simulink model "pmsm_observer_pll_block_model"  (R2024b)
settings: Solver=FixedStepDiscrete  StartTime=0.0  StopTime=0.15  FixedStep=Ts  RelTol=1e-3
InitFcn:
  | model_file = get_param(bdroot, 'FileName');
  | model_dir = fileparts(model_file);
  | run(fullfile(model_dir, 'pmsm_observer_pll_params.m'));
values from neighbouring files (symbols this model uses):
  flux_limit = flux_wb * flux_limit_ratio    (= 0.0117)    [pmsm_observer_pll_params.m]
  flux_wb = 0.0078    [pmsm_observer_pll_params.m]
  Ld = Ls    (= 0.0006)    [pmsm_observer_pll_params.m]
  Lq = Ls    (= 0.0006)    [pmsm_observer_pll_params.m]
  Ls = 0.0006    [pmsm_observer_pll_params.m]
  obs_eps = 1.0e-6    (= 1e-06)    [pmsm_observer_pll_params.m]
  obs_speed_filter_alpha = 0.05    [pmsm_observer_pll_params.m]
  obs_speed_limit_rad_s = 2200.0    (= 2200)    [pmsm_observer_pll_params.m]
  obs_theta_comp_rad = 2.2003    [pmsm_observer_pll_params.m]
  pll_integral_limit = 1800.0    (= 1800)    [pmsm_observer_pll_params.m]
  pll_ki = 3000.0    (= 3000)    [pmsm_observer_pll_params.m]
  pll_kp = 120.0    (= 120)    [pmsm_observer_pll_params.m]
  pole_pairs = 4.0    (= 4)    [pmsm_observer_pll_params.m]
  Rs = 0.53    [pmsm_observer_pll_params.m]
  sim_id_a = 0.0    (= 0)    [pmsm_observer_pll_params.m]
  sim_iq_a = 1.0    (= 1)    [pmsm_observer_pll_params.m]
  sim_mech_speed_rad_s = 2000.0 * 2.0 * pi / 60.0    (= 209.439510239)    [pmsm_observer_pll_params.m]
  Ts = 6.25e-5    (= 6.25e-05)    [pmsm_observer_pll_params.m]
undefined symbols (not defined in the file or in its folder): DiscIntNeverNeededParam
settings Model: Creator=10095  LastModifiedBy=10095
settings DataIOCC: SaveFormat=StructureWithTime

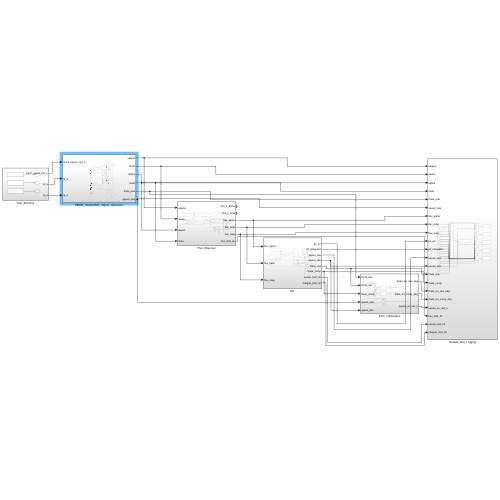
[thumbnail: Simulink's stored preview of the top-level diagram]
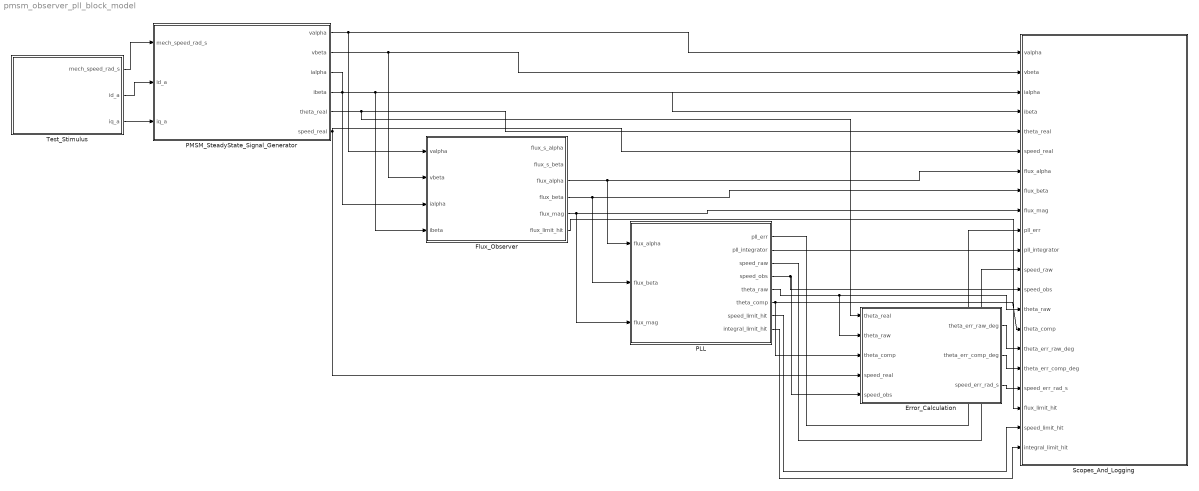
== system pmsm_observer_pll_block_model ==
  Error_Calculation : Subsystem
  Flux_Observer : Subsystem
  PLL : Subsystem
  PMSM_SteadyState_Signal_Generator : Subsystem
  Scopes_And_Logging : Subsystem
  Test_Stimulus : Subsystem
  wires:
  Test_Stimulus/3(iq_a) -> PMSM_SteadyState_Signal_Generator/3(iq_a)
  PLL/6(theta_comp) -> Error_Calculation/3(theta_comp), Scopes_And_Logging/15(theta_comp)
  PLL/2(pll_integrator) -> Scopes_And_Logging/11(pll_integrator)
  Flux_Observer/4(flux_beta) -> Scopes_And_Logging/8(flux_beta), PLL/2(flux_beta)
  Test_Stimulus/1(mech_speed_rad_s) -> PMSM_SteadyState_Signal_Generator/1(mech_speed_rad_s)
  Test_Stimulus/2(id_a) -> PMSM_SteadyState_Signal_Generator/2(id_a)
  PMSM_SteadyState_Signal_Generator/5(theta_real) -> Error_Calculation/1(theta_real), Scopes_And_Logging/5(theta_real)
  PMSM_SteadyState_Signal_Generator/4(ibeta) -> Scopes_And_Logging/4(ibeta), Flux_Observer/4(ibeta)
  PMSM_SteadyState_Signal_Generator/3(ialpha) -> Scopes_And_Logging/3(ialpha), Flux_Observer/3(ialpha)
  Error_Calculation/1(theta_err_raw_deg) -> Scopes_And_Logging/16(theta_err_raw_deg)
  PMSM_SteadyState_Signal_Generator/2(vbeta) -> Scopes_And_Logging/2(vbeta), Flux_Observer/2(vbeta)
  PMSM_SteadyState_Signal_Generator/1(valpha) -> Scopes_And_Logging/1(valpha), Flux_Observer/1(valpha)
  PMSM_SteadyState_Signal_Generator/6(speed_real) -> Error_Calculation/4(speed_real), Scopes_And_Logging/6(speed_real)
  PLL/7(speed_limit_hit) -> Scopes_And_Logging/20(speed_limit_hit)
  PLL/3(speed_raw) -> Scopes_And_Logging/12(speed_raw)
  Flux_Observer/3(flux_alpha) -> Scopes_And_Logging/7(flux_alpha), PLL/1(flux_alpha)
  PLL/5(theta_raw) -> Scopes_And_Logging/14(theta_raw), Error_Calculation/2(theta_raw)
  PLL/1(pll_err) -> Scopes_And_Logging/10(pll_err)
  Flux_Observer/5(flux_mag) -> Scopes_And_Logging/9(flux_mag), PLL/3(flux_mag)
  Flux_Observer/6(flux_limit_hit) -> Scopes_And_Logging/19(flux_limit_hit)
  PLL/4(speed_obs) -> Scopes_And_Logging/13(speed_obs), Error_Calculation/5(speed_obs)
  PLL/8(integral_limit_hit) -> Scopes_And_Logging/21(integral_limit_hit)
  Error_Calculation/2(theta_err_comp_deg) -> Scopes_And_Logging/17(theta_err_comp_deg)
  Error_Calculation/3(speed_err_rad_s) -> Scopes_And_Logging/18(speed_err_rad_s)

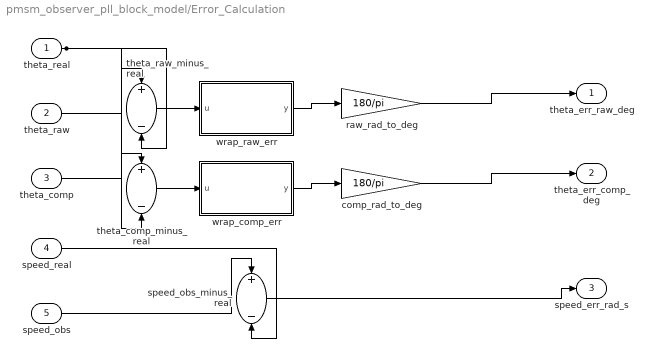
== system pmsm_observer_pll_block_model/Error_Calculation ==
  theta_real : Inport
  theta_raw : Inport  Port=2
  theta_comp : Inport  Port=3
  speed_real : Inport  Port=4
  speed_obs : Inport  Port=5
  comp_rad_to_deg : Gain  Gain=180/pi
  raw_rad_to_deg : Gain  Gain=180/pi
  speed_obs_minus_real : Sum  Inputs=+-
  theta_comp_minus_real : Sum  Inputs=+-
  theta_raw_minus_real : Sum  Inputs=+-
  wrap_comp_err : MATLAB Function  TreatAsAtomicUnit=on
  wrap_raw_err : MATLAB Function  TreatAsAtomicUnit=on
  theta_err_raw_deg : Outport
  theta_err_comp_deg : Outport  Port=2
  speed_err_rad_s : Outport  Port=3
  wires:
  theta_raw/1 -> theta_raw_minus_real/1
  theta_real/1 -> theta_raw_minus_real/2, theta_comp_minus_real/2
  theta_raw_minus_real/1 -> wrap_raw_err/1(u)
  wrap_raw_err/1(y) -> raw_rad_to_deg/1
  raw_rad_to_deg/1 -> theta_err_raw_deg/1
  theta_comp/1 -> theta_comp_minus_real/1
  theta_comp_minus_real/1 -> wrap_comp_err/1(u)
  wrap_comp_err/1(y) -> comp_rad_to_deg/1
  comp_rad_to_deg/1 -> theta_err_comp_deg/1
  speed_obs/1 -> speed_obs_minus_real/1
  speed_real/1 -> speed_obs_minus_real/2
  speed_obs_minus_real/1 -> speed_err_rad_s/1

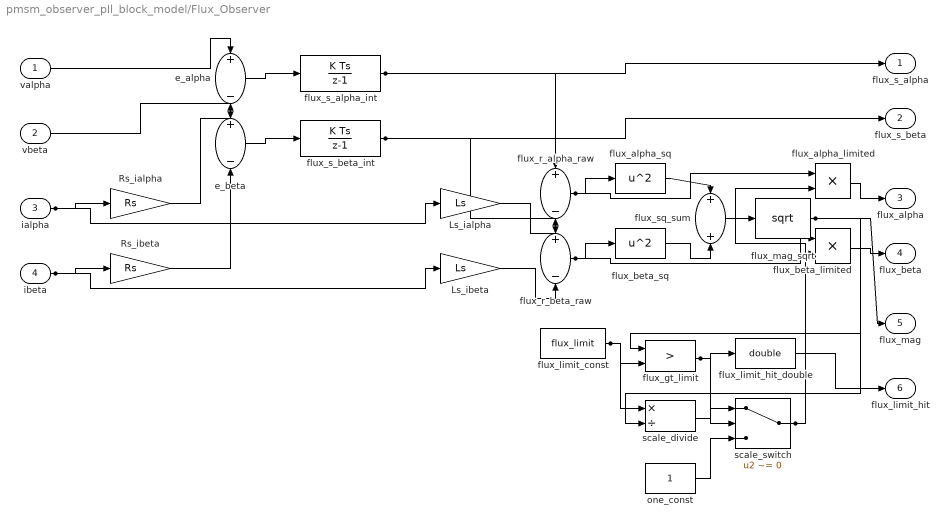
== system pmsm_observer_pll_block_model/Flux_Observer ==
  valpha : Inport
  vbeta : Inport  Port=2
  ialpha : Inport  Port=3
  ibeta : Inport  Port=4
  Ls_ialpha : Gain  Gain=Ls
  Ls_ibeta : Gain  Gain=Ls
  Rs_ialpha : Gain  Gain=Rs
  Rs_ibeta : Gain  Gain=Rs
  e_alpha : Sum  Inputs=+-
  e_beta : Sum  Inputs=+-
  flux_alpha_limited : Product
  flux_alpha_sq : Math  Operator=square
  flux_beta_limited : Product
  flux_beta_sq : Math  Operator=square
  flux_gt_limit : RelationalOperator  Operator=>  OutDataTypeStr=boolean  RndMeth=Simplest  InputSameDT=off
  flux_limit_const : Constant  Value=flux_limit
  flux_limit_hit_double : DataTypeConversion  OutDataTypeStr=double  SaturateOnIntegerOverflow=off  RndMeth=Floor
  flux_mag_sqrt : Math  Operator=sqrt
  flux_r_alpha_raw : Sum  Inputs=+-
  flux_r_beta_raw : Sum  Inputs=+-
  flux_s_alpha_int : DiscreteIntegrator  InitialCondition=flux_wb  SampleTime=Ts  ICPrevOutput=DiscIntNeverNeededParam  ICPrevScaledInput=DiscIntNeverNeededParam
  flux_s_beta_int : DiscreteIntegrator  SampleTime=Ts  ICPrevOutput=DiscIntNeverNeededParam  ICPrevScaledInput=DiscIntNeverNeededParam
  flux_sq_sum : Sum
  one_const : Constant
  scale_divide : Product  Inputs=*/
  scale_switch : Switch  Criteria=u2 ~= 0  SaturateOnIntegerOverflow=off  InputSameDT=off
  flux_s_alpha : Outport
  flux_s_beta : Outport  Port=2
  flux_alpha : Outport  Port=3
  flux_beta : Outport  Port=4
  flux_mag : Outport  Port=5
  flux_limit_hit : Outport  Port=6
  wires:
  ialpha/1 -> Rs_ialpha/1, Ls_ialpha/1
  ibeta/1 -> Rs_ibeta/1, Ls_ibeta/1
  valpha/1 -> e_alpha/1
  Rs_ialpha/1 -> e_alpha/2
  vbeta/1 -> e_beta/1
  Rs_ibeta/1 -> e_beta/2
  e_alpha/1 -> flux_s_alpha_int/1
  e_beta/1 -> flux_s_beta_int/1
  flux_s_alpha_int/1 -> flux_s_alpha/1, flux_r_alpha_raw/1
  flux_s_beta_int/1 -> flux_s_beta/1, flux_r_beta_raw/1
  Ls_ialpha/1 -> flux_r_alpha_raw/2
  Ls_ibeta/1 -> flux_r_beta_raw/2
  flux_r_alpha_raw/1 -> flux_alpha_sq/1, flux_alpha_limited/1
  flux_r_beta_raw/1 -> flux_beta_sq/1, flux_beta_limited/1
  flux_alpha_sq/1 -> flux_sq_sum/1
  flux_beta_sq/1 -> flux_sq_sum/2
  flux_sq_sum/1 -> flux_mag_sqrt/1
  flux_mag_sqrt/1 -> flux_mag/1, flux_gt_limit/1, scale_divide/2
  flux_limit_const/1 -> flux_gt_limit/2, scale_divide/1
  flux_gt_limit/1 -> flux_limit_hit_double/1, scale_switch/2
  flux_limit_hit_double/1 -> flux_limit_hit/1
  scale_divide/1 -> scale_switch/1
  one_const/1 -> scale_switch/3
  scale_switch/1 -> flux_alpha_limited/2, flux_beta_limited/2
  flux_alpha_limited/1 -> flux_alpha/1
  flux_beta_limited/1 -> flux_beta/1

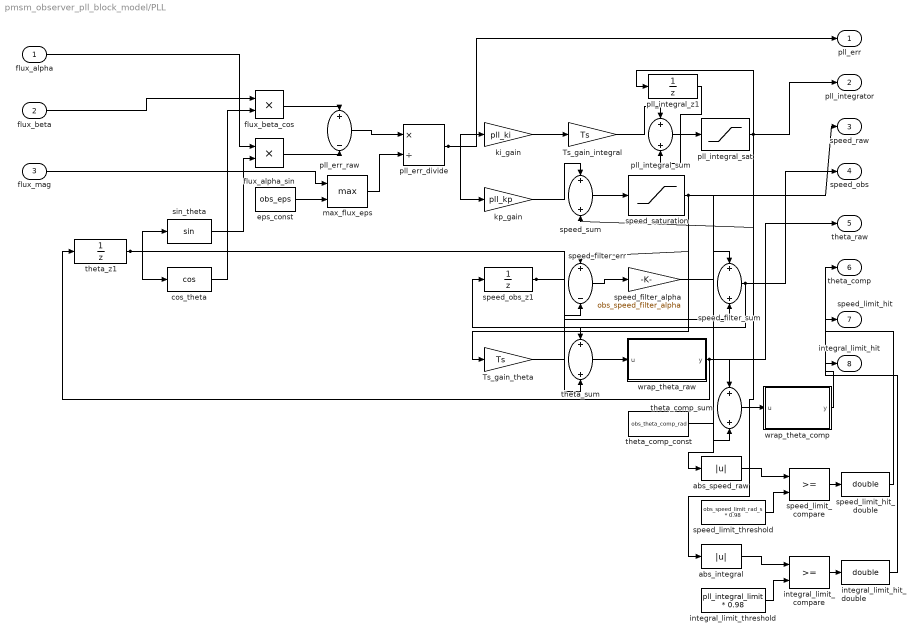
== system pmsm_observer_pll_block_model/PLL ==
  flux_alpha : Inport
  flux_beta : Inport  Port=2
  flux_mag : Inport  Port=3
  Ts_gain_integral : Gain  Gain=Ts
  Ts_gain_theta : Gain  Gain=Ts
  abs_integral : Abs  SaturateOnIntegerOverflow=off
  abs_speed_raw : Abs  SaturateOnIntegerOverflow=off
  cos_theta : Trigonometry  Operator=cos
  eps_const : Constant  Value=obs_eps
  flux_alpha_sin : Product
  flux_beta_cos : Product
  integral_limit_compare : RelationalOperator  OutDataTypeStr=boolean  RndMeth=Simplest  InputSameDT=off
  integral_limit_hit_double : DataTypeConversion  OutDataTypeStr=double  SaturateOnIntegerOverflow=off  RndMeth=Floor
  integral_limit_threshold : Constant  Value=pll_integral_limit * 0.98
  ki_gain : Gain  Gain=pll_ki
  kp_gain : Gain  Gain=pll_kp
  max_flux_eps : MinMax  Function=max  Inputs=2
  pll_err_divide : Product  Inputs=*/
  pll_err_raw : Sum  Inputs=+-
  pll_integral_sat : Saturate  UpperLimit=pll_integral_limit  LowerLimit=-pll_integral_limit
  pll_integral_sum : Sum
  pll_integral_z1 : UnitDelay  SampleTime=Ts  HasFrameUpgradeWarning=on
  sin_theta : Trigonometry
  speed_filter_alpha : Gain  Gain=obs_speed_filter_alpha
  speed_filter_err : Sum  Inputs=+-
  speed_filter_sum : Sum
  speed_limit_compare : RelationalOperator  OutDataTypeStr=boolean  RndMeth=Simplest  InputSameDT=off
  speed_limit_hit_double : DataTypeConversion  OutDataTypeStr=double  SaturateOnIntegerOverflow=off  RndMeth=Floor
  speed_limit_threshold : Constant  Value=obs_speed_limit_rad_s * 0.98
  speed_obs_z1 : UnitDelay  SampleTime=Ts  HasFrameUpgradeWarning=on
  speed_saturation : Saturate  UpperLimit=obs_speed_limit_rad_s  LowerLimit=-obs_speed_limit_rad_s
  speed_sum : Sum
  theta_comp_const : Constant  Value=obs_theta_comp_rad
  theta_comp_sum : Sum
  theta_sum : Sum
  theta_z1 : UnitDelay  SampleTime=Ts  HasFrameUpgradeWarning=on
  wrap_theta_comp : MATLAB Function  TreatAsAtomicUnit=on
  wrap_theta_raw : MATLAB Function  TreatAsAtomicUnit=on
  pll_err : Outport
  pll_integrator : Outport  Port=2
  speed_raw : Outport  Port=3
  speed_obs : Outport  Port=4
  theta_raw : Outport  Port=5
  theta_comp : Outport  Port=6
  speed_limit_hit : Outport  Port=7
  integral_limit_hit : Outport  Port=8
  wires:
  theta_z1/1 -> sin_theta/1, cos_theta/1, theta_sum/2
  flux_beta/1 -> flux_beta_cos/1
  cos_theta/1 -> flux_beta_cos/2
  flux_alpha/1 -> flux_alpha_sin/1
  sin_theta/1 -> flux_alpha_sin/2
  flux_beta_cos/1 -> pll_err_raw/1
  flux_alpha_sin/1 -> pll_err_raw/2
  flux_mag/1 -> max_flux_eps/1
  eps_const/1 -> max_flux_eps/2
  pll_err_raw/1 -> pll_err_divide/1
  max_flux_eps/1 -> pll_err_divide/2
  pll_err_divide/1 -> pll_err/1, ki_gain/1, kp_gain/1
  ki_gain/1 -> Ts_gain_integral/1
  Ts_gain_integral/1 -> pll_integral_sum/1
  pll_integral_z1/1 -> pll_integral_sum/2
  pll_integral_sum/1 -> pll_integral_sat/1
  pll_integral_sat/1 -> pll_integral_z1/1, pll_integrator/1, speed_sum/2, abs_integral/1
  kp_gain/1 -> speed_sum/1
  speed_sum/1 -> speed_saturation/1
  speed_saturation/1 -> speed_raw/1, speed_filter_err/1, Ts_gain_theta/1, abs_speed_raw/1
  speed_obs_z1/1 -> speed_filter_err/2, speed_filter_sum/2
  speed_filter_err/1 -> speed_filter_alpha/1
  speed_filter_alpha/1 -> speed_filter_sum/1
  speed_filter_sum/1 -> speed_obs_z1/1, speed_obs/1
  Ts_gain_theta/1 -> theta_sum/1
  theta_sum/1 -> wrap_theta_raw/1(u)
  wrap_theta_raw/1(y) -> theta_z1/1, theta_raw/1, theta_comp_sum/1
  theta_comp_const/1 -> theta_comp_sum/2
  theta_comp_sum/1 -> wrap_theta_comp/1(u)
  wrap_theta_comp/1(y) -> theta_comp/1
  abs_speed_raw/1 -> speed_limit_compare/1
  speed_limit_threshold/1 -> speed_limit_compare/2
  speed_limit_compare/1 -> speed_limit_hit_double/1
  speed_limit_hit_double/1 -> speed_limit_hit/1
  abs_integral/1 -> integral_limit_compare/1
  integral_limit_threshold/1 -> integral_limit_compare/2
  integral_limit_compare/1 -> integral_limit_hit_double/1
  integral_limit_hit_double/1 -> integral_limit_hit/1

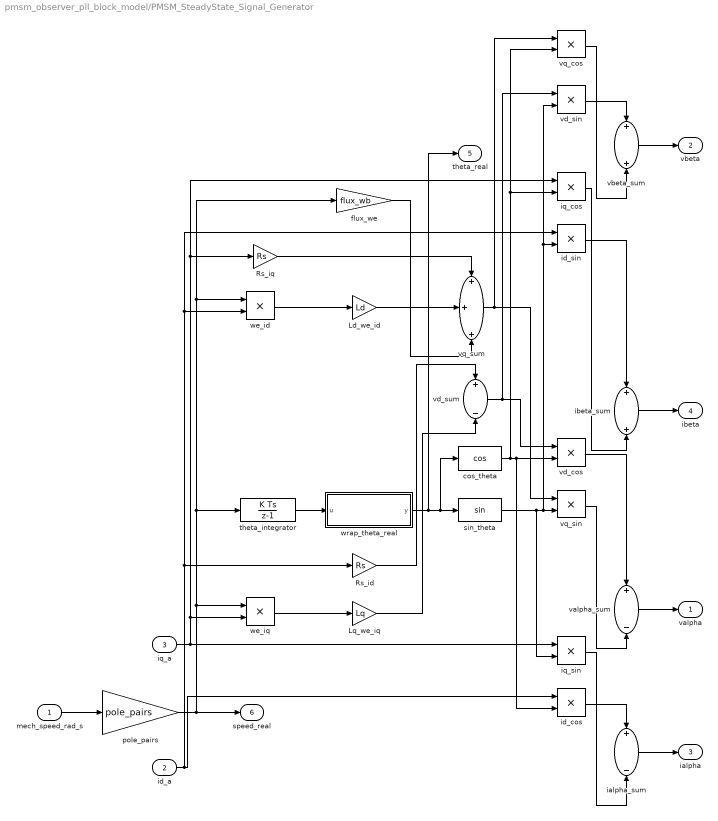
== system pmsm_observer_pll_block_model/PMSM_SteadyState_Signal_Generator ==
  mech_speed_rad_s : Inport
  id_a : Inport  Port=2
  iq_a : Inport  Port=3
  Ld_we_id : Gain  Gain=Ld
  Lq_we_iq : Gain  Gain=Lq
  Rs_id : Gain  Gain=Rs
  Rs_iq : Gain  Gain=Rs
  cos_theta : Trigonometry  Operator=cos
  flux_we : Gain  Gain=flux_wb
  ialpha_sum : Sum  Inputs=+-
  ibeta_sum : Sum
  id_cos : Product
  id_sin : Product
  iq_cos : Product
  iq_sin : Product
  pole_pairs : Gain  Gain=pole_pairs
  sin_theta : Trigonometry
  theta_integrator : DiscreteIntegrator  SampleTime=Ts  ICPrevOutput=DiscIntNeverNeededParam  ICPrevScaledInput=DiscIntNeverNeededParam
  valpha_sum : Sum  Inputs=+-
  vbeta_sum : Sum
  vd_cos : Product
  vd_sin : Product
  vd_sum : Sum  Inputs=+-
  vq_cos : Product
  vq_sin : Product
  vq_sum : Sum  Inputs=+++
  we_id : Product
  we_iq : Product
  wrap_theta_real : MATLAB Function  TreatAsAtomicUnit=on
  valpha : Outport
  vbeta : Outport  Port=2
  ialpha : Outport  Port=3
  ibeta : Outport  Port=4
  theta_real : Outport  Port=5
  speed_real : Outport  Port=6
  wires:
  id_a/1 -> id_sin/1, we_id/2, Rs_id/1, id_cos/1
  iq_a/1 -> Rs_iq/1, iq_cos/1, we_iq/2, iq_sin/1
  mech_speed_rad_s/1 -> pole_pairs/1
  vbeta_sum/1 -> vbeta/1
  vd_sin/1 -> vbeta_sum/1
  theta_integrator/1 -> wrap_theta_real/1(u)
  pole_pairs/1 -> flux_we/1, we_id/1, theta_integrator/1, we_iq/1, speed_real/1
  Rs_iq/1 -> vq_sum/1
  we_iq/1 -> Lq_we_iq/1
  we_id/1 -> Ld_we_id/1
  ibeta_sum/1 -> ibeta/1
  id_sin/1 -> ibeta_sum/1
  flux_we/1 -> vq_sum/3
  Ld_we_id/1 -> vq_sum/2
  vq_sin/1 -> valpha_sum/2
  vd_sum/1 -> vd_cos/1, vd_sin/1
  wrap_theta_real/1(y) -> cos_theta/1, sin_theta/1, theta_real/1
  Rs_id/1 -> vd_sum/1
  ialpha_sum/1 -> ialpha/1
  id_cos/1 -> ialpha_sum/1
  Lq_we_iq/1 -> vd_sum/2
  vq_cos/1 -> vbeta_sum/2
  vq_sum/1 -> vq_sin/1, vq_cos/1
  cos_theta/1 -> id_cos/2, vd_cos/2, iq_cos/2, vq_cos/2
  sin_theta/1 -> id_sin/2, vd_sin/2, vq_sin/2, iq_sin/2
  iq_cos/1 -> ibeta_sum/2
  valpha_sum/1 -> valpha/1
  vd_cos/1 -> valpha_sum/1
  iq_sin/1 -> ialpha_sum/2

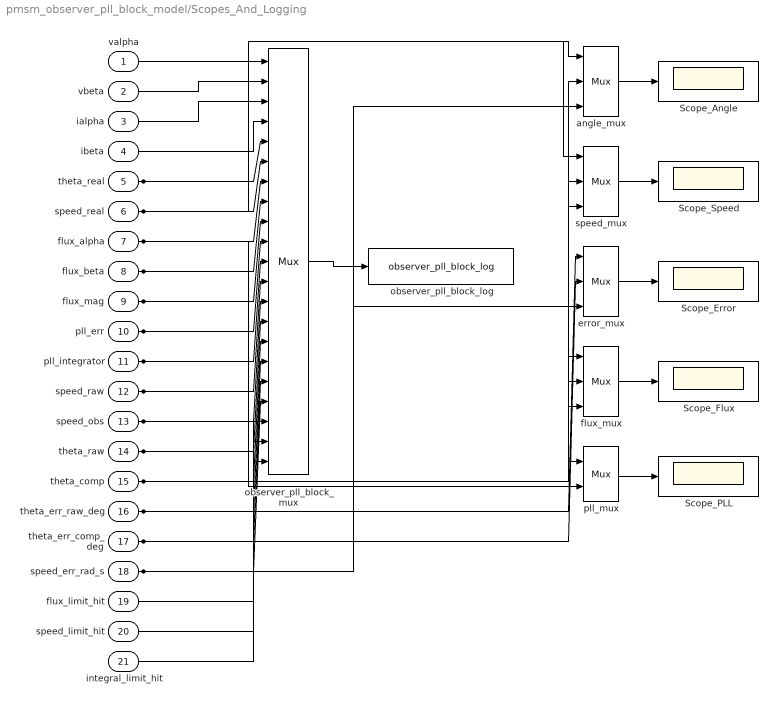
== system pmsm_observer_pll_block_model/Scopes_And_Logging ==
  valpha : Inport
  vbeta : Inport  Port=2
  ialpha : Inport  Port=3
  ibeta : Inport  Port=4
  theta_real : Inport  Port=5
  speed_real : Inport  Port=6
  flux_alpha : Inport  Port=7
  flux_beta : Inport  Port=8
  flux_mag : Inport  Port=9
  pll_err : Inport  Port=10
  pll_integrator : Inport  Port=11
  speed_raw : Inport  Port=12
  speed_obs : Inport  Port=13
  theta_raw : Inport  Port=14
  theta_comp : Inport  Port=15
  theta_err_raw_deg : Inport  Port=16
  theta_err_comp_deg : Inport  Port=17
  speed_err_rad_s : Inport  Port=18
  flux_limit_hit : Inport  Port=19
  speed_limit_hit : Inport  Port=20
  integral_limit_hit : Inport  Port=21
  Scope_Angle : Scope
  Scope_Error : Scope
  Scope_Flux : Scope
  Scope_PLL : Scope
  Scope_Speed : Scope
  angle_mux : Mux  Inputs=3
  error_mux : Mux  Inputs=3
  flux_mux : Mux  Inputs=3
  observer_pll_block_log : ToWorkspace  VariableName=observer_pll_block_log  SampleTime=-1
  observer_pll_block_mux : Mux  Inputs=21
  pll_mux : Mux  Inputs=2
  speed_mux : Mux  Inputs=3
  wires:
  valpha/1 -> observer_pll_block_mux/1
  vbeta/1 -> observer_pll_block_mux/2
  ialpha/1 -> observer_pll_block_mux/3
  ibeta/1 -> observer_pll_block_mux/4
  theta_real/1 -> observer_pll_block_mux/5, angle_mux/1
  speed_real/1 -> observer_pll_block_mux/6, speed_mux/1
  flux_alpha/1 -> observer_pll_block_mux/7, flux_mux/1
  flux_beta/1 -> observer_pll_block_mux/8, flux_mux/2
  flux_mag/1 -> observer_pll_block_mux/9, flux_mux/3
  pll_err/1 -> observer_pll_block_mux/10, pll_mux/1
  pll_integrator/1 -> observer_pll_block_mux/11, pll_mux/2
  speed_raw/1 -> observer_pll_block_mux/12, speed_mux/2
  speed_obs/1 -> observer_pll_block_mux/13, speed_mux/3
  theta_raw/1 -> observer_pll_block_mux/14, angle_mux/2
  theta_comp/1 -> observer_pll_block_mux/15, angle_mux/3
  theta_err_raw_deg/1 -> observer_pll_block_mux/16, error_mux/1
  theta_err_comp_deg/1 -> observer_pll_block_mux/17, error_mux/2
  speed_err_rad_s/1 -> observer_pll_block_mux/18, error_mux/3
  flux_limit_hit/1 -> observer_pll_block_mux/19
  speed_limit_hit/1 -> observer_pll_block_mux/20
  integral_limit_hit/1 -> observer_pll_block_mux/21
  observer_pll_block_mux/1 -> observer_pll_block_log/1
  angle_mux/1 -> Scope_Angle/1
  speed_mux/1 -> Scope_Speed/1
  error_mux/1 -> Scope_Error/1
  flux_mux/1 -> Scope_Flux/1
  pll_mux/1 -> Scope_PLL/1

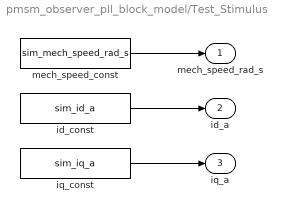
== system pmsm_observer_pll_block_model/Test_Stimulus ==
  id_const : Constant  Value=sim_id_a
  iq_const : Constant  Value=sim_iq_a
  mech_speed_const : Constant  Value=sim_mech_speed_rad_s
  mech_speed_rad_s : Outport
  id_a : Outport  Port=2
  iq_a : Outport  Port=3
  wires:
  mech_speed_const/1 -> mech_speed_rad_s/1
  id_const/1 -> id_a/1
  iq_const/1 -> iq_a/1

== matlab function pmsm_observer_pll_block_model/PMSM_SteadyState_Signal_Generator/wrap_theta_real ==
  data: u input; y output
function y = fcn(u)
%#codegen
y = u - floor(u / 6.283185307179586) * 6.283185307179586;
end

== matlab function pmsm_observer_pll_block_model/PLL/wrap_theta_comp ==
  data: u input; y output
function y = fcn(u)
%#codegen
y = u - floor(u / 6.283185307179586) * 6.283185307179586;
end

== matlab function pmsm_observer_pll_block_model/Error_Calculation/wrap_raw_err ==
  data: u input; y output
function y = fcn(u)
%#codegen
y = u;
while y > 3.141592653589793
    y = y - 6.283185307179586;
end
while y < -3.141592653589793
    y = y + 6.283185307179586;
end
end

== matlab function pmsm_observer_pll_block_model/Error_Calculation/wrap_comp_err ==
  data: u input; y output
function y = fcn(u)
%#codegen
y = u;
while y > 3.141592653589793
    y = y - 6.283185307179586;
end
while y < -3.141592653589793
    y = y + 6.283185307179586;
end
end

== matlab function pmsm_observer_pll_block_model/PLL/wrap_theta_raw ==
  data: u input; y output
function y = fcn(u)
%#codegen
y = u - floor(u / 6.283185307179586) * 6.283185307179586;
end
